simulink model "Two_Attitude_Estimation_ekf"  (R2021a)
settings: Solver=FixedStepAuto  StartTime=0.0  StopTime=200  FixedStep=Ts  RelTol=1e-5
values from neighbouring files (symbols this model uses):
  accel_filter_coef = [    0.0264    0.1405    0.3331    0.3331    0.1405    0.0264]    [quad_params_ekf.m]
  g = ref_acc(3)    [ekf_measurement_jacobian.m]    (also in quad_params_ekf.m = 9.81)
  gyro_filter_den = [ 1.0000    2.2287    2.5245    1.5773    0.5410    0.0796]    [quad_params_ekf.m]
  gyro_filter_num = [ 0.2821    1.2725    2.4208    2.4208    1.2725    0.2821]    [quad_params_ekf.m]
  I = [     0.005831943165131                   0                   0 ... (first row only)    [quad_params_ekf.m]
  Kd_rates = [0.05,0.05,0.1]'    [quad_params_ekf.m]
  Kd_vel = [0.8,0.8,0.3]'    [quad_params_ekf.m]
  Ki_vel = [0.1,0.1,0.1]'    [quad_params_ekf.m]
  km = 1.2e-7    (= 1.2e-07)    [quad_params_ekf.m]
  Kp_att = [6,6,6]'    [quad_params_ekf.m]
  Kp_pos = [7,7,3]'    [quad_params_ekf.m]
  Kp_rates = [10,10,10]'    [quad_params_ekf.m]
  Kp_vel = [3,3,5]'    [quad_params_ekf.m]
  kt = 0.9e-5    (= 9e-06)    [quad_params_ekf.m]
  L = 0.2    [quad_params_ekf.m]
  m = 0.9272    [quad_params_ekf.m]
  P_init = 0.01*eye(7)    [quad_params_ekf.m]
  Q = diag([0.015,0.0150,0.0150,0.0150,0.001,0.001,0.001])    [quad_params_ekf.m]
  q_init = [1;0;0;0]    [quad_params_ekf.m]
  R = diag([0.35,0.35,0.35,0.05,0.05,0.05])    [quad_params_ekf.m]
  rate_p_max = 3.5    [quad_params_ekf.m]
  thrust_max = thrust_max_per_motor*4    (= 32)    [quad_params_ekf.m]
  thrust_max_per_motor = 8    [quad_params_ekf.m]
  tilt_max = pi/6    (= 0.523598775598)    [quad_params_ekf.m]
  TQ_max_per_motor = km*(w_max.^2)    [quad_params_ekf.m]
  Ts = 0.001    [ekf_process_jacobian.m]    (also in ekf_process_model.m; quad_params_ekf.m)
  Ts_IMU = 0.001    [quad_params_ekf.m]
  Vb_init = [0;0;0]    [quad_params_ekf.m]
  vel_xy_max = 15    [quad_params_ekf.m]
  vel_z_max = 10    [quad_params_ekf.m]
  wb_init = [0;0;0]    [quad_params_ekf.m]
  x_0 = [1 0 0 0 0 0 0]'    [quad_params_ekf.m]
  Xe_init = [0;0;0]    [quad_params_ekf.m]
undefined symbols (not defined in the file or in its folder): IMU, p, pm_0, sigbuilder_block, Vm_0, xme_0
libraries: aerolibutil x8, simulink_extras x8, sharedtransform x7, sharedutil x6, simulink x4, pid_lib x3, aerolibcommonsys x3, aerolibnavsys x2, dspstat3 x2, mspsensorlib x1, aerolibnav x1, dspmtrx3 x1
(part 4 of 4)

== system Two_Attitude_Estimation_ekf/Trajectory command/X ramp/ ramp on X ==
  Demux : Demux  Tag=STV Demux
      settings: DisplayOption=none
  FromWs : FromWorkspace  Tag=STV FromWs  VariableName=tuvar
      SigBuilderData=|
      | common.afterFinalStr = 'Extrapolate'
      | common.sampleTime = 0
      | dataSet(1).timeRange = [0 200]
      | dataSet(1).name = 'small_steps'
      | dataSet(2).timeRange = [0 200]
      | dataSet(2).name = 'zStairs_xyConstVEL'
      | dataSet(3).timeRange = [0 500]
      | dataSet(3).name = 'sineWaves'
      | dataSet(4).timeRange = [0 200]
      | dataSet(4).name = 'ZERO'
      | dataSet(5).timeRange = [0 5]
      | dataSet(5).name = 'SEARCH_P1'
      | sbobj.Name = 'Signal Builder'
      | sbobj.Groups(1).Name = 'small_steps'
      | sbobj.Groups(1).Signals(1).Name = 'Z'
      | sbobj.Groups(1).Signals(1).XData = [0 10 10.000001 20 20.000001 30 30.000001 55 200]
      | sbobj.Groups(1).Signals(1).YData = [0 0 2 2 2 2 2 2 2]
      | sbobj.Groups(1).Signals(2).Name = 'Y'
      | sbobj.Groups(1).Signals(2).XData = [0 10 10.000001 20 20.000001 30 30.000001 55 200]
      | sbobj.Groups(1).Signals(2).YData = [0 0 0 0 3 3 3 3 3]
      | sbobj.Groups(1).Signals(3).Name = 'X'
      | sbobj.Groups(1).Signals(3).XData = [0 10 10.000001 20 20.000001 30 30.000001 55 200]
      | sbobj.Groups(1).Signals(3).YData = [0 0 0 0 0 0 1 1 1]
      | sbobj.Groups(1).Signals(4).Name = 'Yaw'
      | sbobj.Groups(1).Signals(4).XData = [0 200]
      | sbobj.Groups(1).Signals(4).YData = [0 0]
      | sbobj.Groups(1).TimeRange = [0 200]
      | sbobj.Groups(2).Name = 'zStairs_xyConstVEL'
      | sbobj.Groups(2).Signals(1).Name = 'Z'
      | sbobj.Groups(2).Signals(1).XData = [0 10 10.000001 20 20.000001 30 30.000001 40 40.000001 55 200]
      | sbobj.Groups(2).Signals(1).YData = [0 0 1 1 2 2 1 1 0 0 0]
      | sbobj.Groups(2).Signals(2).Name = 'Y'
      | sbobj.Groups(2).Signals(2).XData = [0 10 10.000001 20 20.000001 30 30.000001 40 40.000001 55 200]
      | sbobj.Groups(2).Signals(2).YData = [0 1 1.0000001 2 2.0000001 3 3.0000001 4 4.0000001 5.5 20]
      | sbobj.Groups(2).Signals(3).Name = 'X'
      | sbobj.Groups(2).Signals(3).XData = [0 10 10.000001 20 20.000001 30 30.000001 40 40.000001 55 200]
      | sbobj.Groups(2).Signals(3).YData = [0 0.5 0.50000005 1 1.00000005 1.5 1.50000005 2 2.00000005 2.75 10]
      | sbobj.Groups(2).Signals(4).Name = 'Yaw'
      | sbobj.Groups(2).Signals(4).XData = [0 200]
      | sbobj.Groups(2).Signals(4).YData = [0 0]
      | sbobj.Groups(2).TimeRange = [0 200]
      | sbobj.Groups(3).Name = 'sineWaves'
      | sbobj.Groups(3).Signals(1).Name = 'Z'
      | sbobj.Groups(3).Signals(1).XData = [0 0.1 0.2 0.3 0.4 0.5 0.6 0.7 0.8 0.9 1 1.1 ... (5001 elements, 1x5001)]
      | sbobj.Groups(3).Signals(1).YData = [0 0.0314107325553 0.0627904665622 0.0941082340641 0.125333128258 0.156434333994 0.18738115819 0.218143060119 0.248689681547 0.278990876699 0.309016742004 0.338737645607 ... (5001 elements, 1x5001)]
      | sbobj.Groups(3).Signals(2).Name = 'Y'
      | sbobj.Groups(3).Signals(2).XData = [0 0.1 0.2 0.3 0.4 0.5 0.6 0.7 0.8 0.9 1 1.1 ... (5001 elements, 1x5001)]
      | sbobj.Groups(3).Signals(2).YData = [0 0.01 0.02 0.03 0.04 0.05 0.06 0.07 0.08 0.09 0.1 0.11 ... (5001 elements, 1x5001)]
      | sbobj.Groups(3).Signals(3).Name = 'X'
      | sbobj.Groups(3).Signals(3).XData = [0 0.1 0.2 0.3 0.4 0.5 0.6 0.7 0.8 0.9 1 1.1 ... (5001 elements, 1x5001)]
      | sbobj.Groups(3).Signals(3).YData = [0 0.0157073040455 0.0314107325553 0.04710641095 0.0627904665622 0.0784590295926 0.0941082340641 0.109734218776 0.125333128258 0.140901113717 0.156434333994 0.171928956505 ... (5001 elements, 1x5001)]
      | sbobj.Groups(3).Signals(4).Name = 'Yaw'
      | sbobj.Groups(3).Signals(4).XData = [0 500]
      | sbobj.Groups(3).Signals(4).YData = [0 0]
      | sbobj.Groups(3).TimeRange = [0 500]
      | sbobj.Groups(4).Name = 'ZERO'
      | sbobj.Groups(4).Signals(1).Name = 'Z'
      | sbobj.Groups(4).Signals(1).XData = [0 200]
      | sbobj.Groups(4).Signals(1).YData = [0 0]
      | sbobj.Groups(4).Signals(2).Name = 'Y'
      | sbobj.Groups(4).Signals(2).XData = [0 200]
      | sbobj.Groups(4).Signals(2).YData = [0 0]
      | sbobj.Groups(4).Signals(3).Name = 'X'
      | sbobj.Groups(4).Signals(3).XData = [0 200]
      | sbobj.Groups(4).Signals(3).YData = [0 0]
      | sbobj.Groups(4).Signals(4).Name = 'Yaw'
      | sbobj.Groups(4).Signals(4).XData = [0 200]
      | sbobj.Groups(4).Signals(4).YData = [0 0]
      | sbobj.Groups(4).TimeRange = [0 200]
      | sbobj.Groups(5).Name = 'SEARCH_P1'
      | sbobj.Groups(5).Signals(1).Name = 'Z'
      | sbobj.Groups(5).Signals(1).XData = [0 5]
      | sbobj.Groups(5).Signals(1).YData = [0 0]
      | sbobj.Groups(5).Signals(2).Name = 'Y'
      | sbobj.Groups(5).Signals(2).XData = [0 5]
      | sbobj.Groups(5).Signals(2).YData = [0 0]
      | sbobj.Groups(5).Signals(3).Name = 'X'
      | sbobj.Groups(5).Signals(3).XData = [0 0.2 2 3 5]
      | sbobj.Groups(5).Signals(3).YData = [0 0 1 1 0]
      | sbobj.Groups(5).Signals(4).Name = 'Yaw'
      | sbobj.Groups(5).Signals(4).XData = [0 5]
      | sbobj.Groups(5).Signals(4).YData = [0 0]
      | sbobj.Groups(5).TimeRange = [0 5]
  Z : Outport  VectorParamsAs1DForOutWhenUnconnected=off
  Y : Outport  Tag=STV Outport  Port=2  VectorParamsAs1DForOutWhenUnconnected=off
  X : Outport  Tag=STV Outport  Port=3  VectorParamsAs1DForOutWhenUnconnected=off
  Yaw : Outport  Tag=STV Outport  Port=4
  wires:
  Demux/4 -> Yaw/1
  Demux/3 -> X/1
  Demux/2 -> Y/1
  FromWs/1 -> Demux/1
  Demux/1 -> Z/1

== system Two_Attitude_Estimation_ekf/Trajectory command/X square/sine wave on X ==
  Demux : Demux  Tag=STV Demux
      settings: DisplayOption=none
  FromWs : FromWorkspace  Tag=STV FromWs  VariableName=tuvar
      SigBuilderData=|
      | common.afterFinalStr = 'Extrapolate'
      | common.sampleTime = 0
      | dataSet(1).timeRange = [0 200]
      | dataSet(1).name = 'small_steps'
      | dataSet(2).timeRange = [0 200]
      | dataSet(2).name = 'zStairs_xyConstVEL'
      | dataSet(3).timeRange = [0 500]
      | dataSet(3).name = 'sineWaves'
      | dataSet(4).timeRange = [0 200]
      | dataSet(4).name = 'ZERO'
      | dataSet(5).timeRange = [0 20]
      | dataSet(5).name = 'SEARCH_P1'
      | sbobj.Name = 'Signal Builder'
      | sbobj.Groups(1).Name = 'small_steps'
      | sbobj.Groups(1).Signals(1).Name = 'Z'
      | sbobj.Groups(1).Signals(1).XData = [0 10 10.000001 20 20.000001 30 30.000001 55 200]
      | sbobj.Groups(1).Signals(1).YData = [0 0 2 2 2 2 2 2 2]
      | sbobj.Groups(1).Signals(2).Name = 'Y'
      | sbobj.Groups(1).Signals(2).XData = [0 10 10.000001 20 20.000001 30 30.000001 55 200]
      | sbobj.Groups(1).Signals(2).YData = [0 0 0 0 3 3 3 3 3]
      | sbobj.Groups(1).Signals(3).Name = 'X'
      | sbobj.Groups(1).Signals(3).XData = [0 10 10.000001 20 20.000001 30 30.000001 55 200]
      | sbobj.Groups(1).Signals(3).YData = [0 0 0 0 0 0 1 1 1]
      | sbobj.Groups(1).Signals(4).Name = 'Yaw'
      | sbobj.Groups(1).Signals(4).XData = [0 200]
      | sbobj.Groups(1).Signals(4).YData = [0 0]
      | sbobj.Groups(1).TimeRange = [0 200]
      | sbobj.Groups(2).Name = 'zStairs_xyConstVEL'
      | sbobj.Groups(2).Signals(1).Name = 'Z'
      | sbobj.Groups(2).Signals(1).XData = [0 10 10.000001 20 20.000001 30 30.000001 40 40.000001 55 200]
      | sbobj.Groups(2).Signals(1).YData = [0 0 1 1 2 2 1 1 0 0 0]
      | sbobj.Groups(2).Signals(2).Name = 'Y'
      | sbobj.Groups(2).Signals(2).XData = [0 10 10.000001 20 20.000001 30 30.000001 40 40.000001 55 200]
      | sbobj.Groups(2).Signals(2).YData = [0 1 1.0000001 2 2.0000001 3 3.0000001 4 4.0000001 5.5 20]
      | sbobj.Groups(2).Signals(3).Name = 'X'
      | sbobj.Groups(2).Signals(3).XData = [0 10 10.000001 20 20.000001 30 30.000001 40 40.000001 55 200]
      | sbobj.Groups(2).Signals(3).YData = [0 0.5 0.50000005 1 1.00000005 1.5 1.50000005 2 2.00000005 2.75 10]
      | sbobj.Groups(2).Signals(4).Name = 'Yaw'
      | sbobj.Groups(2).Signals(4).XData = [0 200]
      | sbobj.Groups(2).Signals(4).YData = [0 0]
      | sbobj.Groups(2).TimeRange = [0 200]
      | sbobj.Groups(3).Name = 'sineWaves'
      | sbobj.Groups(3).Signals(1).Name = 'Z'
      | sbobj.Groups(3).Signals(1).XData = [0 0.1 0.2 0.3 0.4 0.5 0.6 0.7 0.8 0.9 1 1.1 ... (5001 elements, 1x5001)]
      | sbobj.Groups(3).Signals(1).YData = [0 0.0314107325553 0.0627904665622 0.0941082340641 0.125333128258 0.156434333994 0.18738115819 0.218143060119 0.248689681547 0.278990876699 0.309016742004 0.338737645607 ... (5001 elements, 1x5001)]
      | sbobj.Groups(3).Signals(2).Name = 'Y'
      | sbobj.Groups(3).Signals(2).XData = [0 0.1 0.2 0.3 0.4 0.5 0.6 0.7 0.8 0.9 1 1.1 ... (5001 elements, 1x5001)]
      | sbobj.Groups(3).Signals(2).YData = [0 0.01 0.02 0.03 0.04 0.05 0.06 0.07 0.08 0.09 0.1 0.11 ... (5001 elements, 1x5001)]
      | sbobj.Groups(3).Signals(3).Name = 'X'
      | sbobj.Groups(3).Signals(3).XData = [0 0.1 0.2 0.3 0.4 0.5 0.6 0.7 0.8 0.9 1 1.1 ... (5001 elements, 1x5001)]
      | sbobj.Groups(3).Signals(3).YData = [0 0.0157073040455 0.0314107325553 0.04710641095 0.0627904665622 0.0784590295926 0.0941082340641 0.109734218776 0.125333128258 0.140901113717 0.156434333994 0.171928956505 ... (5001 elements, 1x5001)]
      | sbobj.Groups(3).Signals(4).Name = 'Yaw'
      | sbobj.Groups(3).Signals(4).XData = [0 500]
      | sbobj.Groups(3).Signals(4).YData = [0 0]
      | sbobj.Groups(3).TimeRange = [0 500]
      | sbobj.Groups(4).Name = 'ZERO'
      | sbobj.Groups(4).Signals(1).Name = 'Z'
      | sbobj.Groups(4).Signals(1).XData = [0 200]
      | sbobj.Groups(4).Signals(1).YData = [0 0]
      | sbobj.Groups(4).Signals(2).Name = 'Y'
      | sbobj.Groups(4).Signals(2).XData = [0 200]
      | sbobj.Groups(4).Signals(2).YData = [0 0]
      | sbobj.Groups(4).Signals(3).Name = 'X'
      | sbobj.Groups(4).Signals(3).XData = [0 200]
      | sbobj.Groups(4).Signals(3).YData = [0 0]
      | sbobj.Groups(4).Signals(4).Name = 'Yaw'
      | sbobj.Groups(4).Signals(4).XData = [0 200]
      | sbobj.Groups(4).Signals(4).YData = [0 0]
      | sbobj.Groups(4).TimeRange = [0 200]
      | sbobj.Groups(5).Name = 'SEARCH_P1'
      | sbobj.Groups(5).Signals(1).Name = 'Z'
      | sbobj.Groups(5).Signals(1).XData = [0 9.9 20]
      | sbobj.Groups(5).Signals(1).YData = [0 0 0]
      | sbobj.Groups(5).Signals(2).Name = 'Y'
      | sbobj.Groups(5).Signals(2).XData = [0 20]
      | sbobj.Groups(5).Signals(2).YData = [0 0]
      | sbobj.Groups(5).Signals(3).Name = 'X'
      | sbobj.Groups(5).Signals(3).XData = [0 5 5 10 10 15 15 20]
      | sbobj.Groups(5).Signals(3).YData = [0.2 0.2 -0.2 -0.2 0.2 0.2 -0.2 -0.2]
      | sbobj.Groups(5).Signals(4).Name = 'Yaw'
      | sbobj.Groups(5).Signals(4).XData = [0 20]
      | sbobj.Groups(5).Signals(4).YData = [0 0]
      | sbobj.Groups(5).TimeRange = [0 20]
  Z : Outport  VectorParamsAs1DForOutWhenUnconnected=off
  Y : Outport  Tag=STV Outport  Port=2  VectorParamsAs1DForOutWhenUnconnected=off
  X : Outport  Tag=STV Outport  Port=3  VectorParamsAs1DForOutWhenUnconnected=off
  Yaw : Outport  Tag=STV Outport  Port=4
  wires:
  Demux/4 -> Yaw/1
  Demux/3 -> X/1
  Demux/2 -> Y/1
  FromWs/1 -> Demux/1
  Demux/1 -> Z/1

== system Two_Attitude_Estimation_ekf/Trajectory command/Y Sine/sine wave on Y ==
  Demux : Demux  Tag=STV Demux
      settings: DisplayOption=none
  FromWs : FromWorkspace  Tag=STV FromWs  VariableName=tuvar
      SigBuilderData=|
      | common.afterFinalStr = 'Extrapolate'
      | common.sampleTime = 0
      | dataSet(1).timeRange = [0 200]
      | dataSet(1).name = 'small_steps'
      | dataSet(2).timeRange = [0 200]
      | dataSet(2).name = 'zStairs_xyConstVEL'
      | dataSet(3).timeRange = [0 500]
      | dataSet(3).name = 'sineWaves'
      | dataSet(4).timeRange = [0 200]
      | dataSet(4).name = 'ZERO'
      | dataSet(5).timeRange = [0 200]
      | dataSet(5).name = 'SEARCH_P1'
      | sbobj.Name = 'Signal Builder'
      | sbobj.Groups(1).Name = 'small_steps'
      | sbobj.Groups(1).Signals(1).Name = 'Z'
      | sbobj.Groups(1).Signals(1).XData = [0 10 10.000001 20 20.000001 30 30.000001 55 200]
      | sbobj.Groups(1).Signals(1).YData = [0 0 2 2 2 2 2 2 2]
      | sbobj.Groups(1).Signals(2).Name = 'Y'
      | sbobj.Groups(1).Signals(2).XData = [0 10 10.000001 20 20.000001 30 30.000001 55 200]
      | sbobj.Groups(1).Signals(2).YData = [0 0 0 0 3 3 3 3 3]
      | sbobj.Groups(1).Signals(3).Name = 'X'
      | sbobj.Groups(1).Signals(3).XData = [0 10 10.000001 20 20.000001 30 30.000001 55 200]
      | sbobj.Groups(1).Signals(3).YData = [0 0 0 0 0 0 1 1 1]
      | sbobj.Groups(1).Signals(4).Name = 'Yaw'
      | sbobj.Groups(1).Signals(4).XData = [0 200]
      | sbobj.Groups(1).Signals(4).YData = [0 0]
      | sbobj.Groups(1).TimeRange = [0 200]
      | sbobj.Groups(2).Name = 'zStairs_xyConstVEL'
      | sbobj.Groups(2).Signals(1).Name = 'Z'
      | sbobj.Groups(2).Signals(1).XData = [0 10 10.000001 20 20.000001 30 30.000001 40 40.000001 55 200]
      | sbobj.Groups(2).Signals(1).YData = [0 0 1 1 2 2 1 1 0 0 0]
      | sbobj.Groups(2).Signals(2).Name = 'Y'
      | sbobj.Groups(2).Signals(2).XData = [0 10 10.000001 20 20.000001 30 30.000001 40 40.000001 55 200]
      | sbobj.Groups(2).Signals(2).YData = [0 1 1.0000001 2 2.0000001 3 3.0000001 4 4.0000001 5.5 20]
      | sbobj.Groups(2).Signals(3).Name = 'X'
      | sbobj.Groups(2).Signals(3).XData = [0 10 10.000001 20 20.000001 30 30.000001 40 40.000001 55 200]
      | sbobj.Groups(2).Signals(3).YData = [0 0.5 0.50000005 1 1.00000005 1.5 1.50000005 2 2.00000005 2.75 10]
      | sbobj.Groups(2).Signals(4).Name = 'Yaw'
      | sbobj.Groups(2).Signals(4).XData = [0 200]
      | sbobj.Groups(2).Signals(4).YData = [0 0]
      | sbobj.Groups(2).TimeRange = [0 200]
      | sbobj.Groups(3).Name = 'sineWaves'
      | sbobj.Groups(3).Signals(1).Name = 'Z'
      | sbobj.Groups(3).Signals(1).XData = [0 0.1 0.2 0.3 0.4 0.5 0.6 0.7 0.8 0.9 1 1.1 ... (5001 elements, 1x5001)]
      | sbobj.Groups(3).Signals(1).YData = [0 0.0314107325553 0.0627904665622 0.0941082340641 0.125333128258 0.156434333994 0.18738115819 0.218143060119 0.248689681547 0.278990876699 0.309016742004 0.338737645607 ... (5001 elements, 1x5001)]
      | sbobj.Groups(3).Signals(2).Name = 'Y'
      | sbobj.Groups(3).Signals(2).XData = [0 0.1 0.2 0.3 0.4 0.5 0.6 0.7 0.8 0.9 1 1.1 ... (5001 elements, 1x5001)]
      | sbobj.Groups(3).Signals(2).YData = [0 0.01 0.02 0.03 0.04 0.05 0.06 0.07 0.08 0.09 0.1 0.11 ... (5001 elements, 1x5001)]
      | sbobj.Groups(3).Signals(3).Name = 'X'
      | sbobj.Groups(3).Signals(3).XData = [0 0.1 0.2 0.3 0.4 0.5 0.6 0.7 0.8 0.9 1 1.1 ... (5001 elements, 1x5001)]
      | sbobj.Groups(3).Signals(3).YData = [0 0.0157073040455 0.0314107325553 0.04710641095 0.0627904665622 0.0784590295926 0.0941082340641 0.109734218776 0.125333128258 0.140901113717 0.156434333994 0.171928956505 ... (5001 elements, 1x5001)]
      | sbobj.Groups(3).Signals(4).Name = 'Yaw'
      | sbobj.Groups(3).Signals(4).XData = [0 500]
      | sbobj.Groups(3).Signals(4).YData = [0 0]
      | sbobj.Groups(3).TimeRange = [0 500]
      | sbobj.Groups(4).Name = 'ZERO'
      | sbobj.Groups(4).Signals(1).Name = 'Z'
      | sbobj.Groups(4).Signals(1).XData = [0 200]
      | sbobj.Groups(4).Signals(1).YData = [0 0]
      | sbobj.Groups(4).Signals(2).Name = 'Y'
      | sbobj.Groups(4).Signals(2).XData = [0 200]
      | sbobj.Groups(4).Signals(2).YData = [0 0]
      | sbobj.Groups(4).Signals(3).Name = 'X'
      | sbobj.Groups(4).Signals(3).XData = [0 200]
      | sbobj.Groups(4).Signals(3).YData = [0 0]
      | sbobj.Groups(4).Signals(4).Name = 'Yaw'
      | sbobj.Groups(4).Signals(4).XData = [0 200]
      | sbobj.Groups(4).Signals(4).YData = [0 0]
      | sbobj.Groups(4).TimeRange = [0 200]
      | sbobj.Groups(5).Name = 'SEARCH_P1'
      | sbobj.Groups(5).Signals(1).Name = 'Z'
      | sbobj.Groups(5).Signals(1).XData = [0 9.9 200]
      | sbobj.Groups(5).Signals(1).YData = [0 0 0]
      | sbobj.Groups(5).Signals(2).Name = 'Y'
      | sbobj.Groups(5).Signals(2).XData = [0 0.689655172414 1.37931034483 2.06896551724 2.75862068966 3.44827586207 4.13793103448 4.8275862069 5.51724137931 6.20689655172 6.89655172414 7.58620689655 ... (291 elements, 1x291)]
      | sbobj.Groups(5).Signals(2).YData = [0 0.214970440211 0.41988910156 0.605174215194 0.762162055128 0.883512044446 0.963549992519 0.998533413851 0.986826522542 0.928976719817 0.827688998157 0.687699458853 ... (291 elements, 1x291)]
      | sbobj.Groups(5).Signals(3).Name = 'X'
      | sbobj.Groups(5).Signals(3).XData = [0 9.9 200]
      | sbobj.Groups(5).Signals(3).YData = [0 0 0]
      | sbobj.Groups(5).Signals(4).Name = 'Yaw'
      | sbobj.Groups(5).Signals(4).XData = [0 200]
      | sbobj.Groups(5).Signals(4).YData = [0 0]
      | sbobj.Groups(5).TimeRange = [0 200]
  Z : Outport  VectorParamsAs1DForOutWhenUnconnected=off
  Y : Outport  Tag=STV Outport  Port=2  VectorParamsAs1DForOutWhenUnconnected=off
  X : Outport  Tag=STV Outport  Port=3  VectorParamsAs1DForOutWhenUnconnected=off
  Yaw : Outport  Tag=STV Outport  Port=4
  wires:
  Demux/4 -> Yaw/1
  Demux/3 -> X/1
  Demux/2 -> Y/1
  FromWs/1 -> Demux/1
  Demux/1 -> Z/1

== system Two_Attitude_Estimation_ekf/Trajectory command/Y ramp/square on Y ==
  Demux : Demux  Tag=STV Demux
      settings: DisplayOption=none
  FromWs : FromWorkspace  Tag=STV FromWs  VariableName=tuvar
      SigBuilderData=|
      | common.afterFinalStr = 'Extrapolate'
      | common.sampleTime = 0
      | dataSet(1).timeRange = [0 200]
      | dataSet(1).name = 'small_steps'
      | dataSet(2).timeRange = [0 200]
      | dataSet(2).name = 'zStairs_xyConstVEL'
      | dataSet(3).timeRange = [0 500]
      | dataSet(3).name = 'sineWaves'
      | dataSet(4).timeRange = [0 200]
      | dataSet(4).name = 'ZERO'
      | dataSet(5).timeRange = [0 20]
      | dataSet(5).name = 'SEARCH_P1'
      | sbobj.Name = 'Signal Builder'
      | sbobj.Groups(1).Name = 'small_steps'
      | sbobj.Groups(1).Signals(1).Name = 'Z'
      | sbobj.Groups(1).Signals(1).XData = [0 10 10.000001 20 20.000001 30 30.000001 55 200]
      | sbobj.Groups(1).Signals(1).YData = [0 0 2 2 2 2 2 2 2]
      | sbobj.Groups(1).Signals(2).Name = 'Y'
      | sbobj.Groups(1).Signals(2).XData = [0 10 10.000001 20 20.000001 30 30.000001 55 200]
      | sbobj.Groups(1).Signals(2).YData = [0 0 0 0 3 3 3 3 3]
      | sbobj.Groups(1).Signals(3).Name = 'X'
      | sbobj.Groups(1).Signals(3).XData = [0 10 10.000001 20 20.000001 30 30.000001 55 200]
      | sbobj.Groups(1).Signals(3).YData = [0 0 0 0 0 0 1 1 1]
      | sbobj.Groups(1).Signals(4).Name = 'Yaw'
      | sbobj.Groups(1).Signals(4).XData = [0 200]
      | sbobj.Groups(1).Signals(4).YData = [0 0]
      | sbobj.Groups(1).TimeRange = [0 200]
      | sbobj.Groups(2).Name = 'zStairs_xyConstVEL'
      | sbobj.Groups(2).Signals(1).Name = 'Z'
      | sbobj.Groups(2).Signals(1).XData = [0 10 10.000001 20 20.000001 30 30.000001 40 40.000001 55 200]
      | sbobj.Groups(2).Signals(1).YData = [0 0 1 1 2 2 1 1 0 0 0]
      | sbobj.Groups(2).Signals(2).Name = 'Y'
      | sbobj.Groups(2).Signals(2).XData = [0 10 10.000001 20 20.000001 30 30.000001 40 40.000001 55 200]
      | sbobj.Groups(2).Signals(2).YData = [0 1 1.0000001 2 2.0000001 3 3.0000001 4 4.0000001 5.5 20]
      | sbobj.Groups(2).Signals(3).Name = 'X'
      | sbobj.Groups(2).Signals(3).XData = [0 10 10.000001 20 20.000001 30 30.000001 40 40.000001 55 200]
      | sbobj.Groups(2).Signals(3).YData = [0 0.5 0.50000005 1 1.00000005 1.5 1.50000005 2 2.00000005 2.75 10]
      | sbobj.Groups(2).Signals(4).Name = 'Yaw'
      | sbobj.Groups(2).Signals(4).XData = [0 200]
      | sbobj.Groups(2).Signals(4).YData = [0 0]
      | sbobj.Groups(2).TimeRange = [0 200]
      | sbobj.Groups(3).Name = 'sineWaves'
      | sbobj.Groups(3).Signals(1).Name = 'Z'
      | sbobj.Groups(3).Signals(1).XData = [0 0.1 0.2 0.3 0.4 0.5 0.6 0.7 0.8 0.9 1 1.1 ... (5001 elements, 1x5001)]
      | sbobj.Groups(3).Signals(1).YData = [0 0.0314107325553 0.0627904665622 0.0941082340641 0.125333128258 0.156434333994 0.18738115819 0.218143060119 0.248689681547 0.278990876699 0.309016742004 0.338737645607 ... (5001 elements, 1x5001)]
      | sbobj.Groups(3).Signals(2).Name = 'Y'
      | sbobj.Groups(3).Signals(2).XData = [0 0.1 0.2 0.3 0.4 0.5 0.6 0.7 0.8 0.9 1 1.1 ... (5001 elements, 1x5001)]
      | sbobj.Groups(3).Signals(2).YData = [0 0.01 0.02 0.03 0.04 0.05 0.06 0.07 0.08 0.09 0.1 0.11 ... (5001 elements, 1x5001)]
      | sbobj.Groups(3).Signals(3).Name = 'X'
      | sbobj.Groups(3).Signals(3).XData = [0 0.1 0.2 0.3 0.4 0.5 0.6 0.7 0.8 0.9 1 1.1 ... (5001 elements, 1x5001)]
      | sbobj.Groups(3).Signals(3).YData = [0 0.0157073040455 0.0314107325553 0.04710641095 0.0627904665622 0.0784590295926 0.0941082340641 0.109734218776 0.125333128258 0.140901113717 0.156434333994 0.171928956505 ... (5001 elements, 1x5001)]
      | sbobj.Groups(3).Signals(4).Name = 'Yaw'
      | sbobj.Groups(3).Signals(4).XData = [0 500]
      | sbobj.Groups(3).Signals(4).YData = [0 0]
      | sbobj.Groups(3).TimeRange = [0 500]
      | sbobj.Groups(4).Name = 'ZERO'
      | sbobj.Groups(4).Signals(1).Name = 'Z'
      | sbobj.Groups(4).Signals(1).XData = [0 200]
      | sbobj.Groups(4).Signals(1).YData = [0 0]
      | sbobj.Groups(4).Signals(2).Name = 'Y'
      | sbobj.Groups(4).Signals(2).XData = [0 200]
      | sbobj.Groups(4).Signals(2).YData = [0 0]
      | sbobj.Groups(4).Signals(3).Name = 'X'
      | sbobj.Groups(4).Signals(3).XData = [0 200]
      | sbobj.Groups(4).Signals(3).YData = [0 0]
      | sbobj.Groups(4).Signals(4).Name = 'Yaw'
      | sbobj.Groups(4).Signals(4).XData = [0 200]
      | sbobj.Groups(4).Signals(4).YData = [0 0]
      | sbobj.Groups(4).TimeRange = [0 200]
      | sbobj.Groups(5).Name = 'SEARCH_P1'
      | sbobj.Groups(5).Signals(1).Name = 'Z'
      | sbobj.Groups(5).Signals(1).XData = [0 9.9 20]
      | sbobj.Groups(5).Signals(1).YData = [0 0 0]
      | sbobj.Groups(5).Signals(2).Name = 'Y'
      | sbobj.Groups(5).Signals(2).XData = [0 5 7 10 12 15 17 20]
      | sbobj.Groups(5).Signals(2).YData = [0.2 0.2 -0.2 -0.2 0.2 0.2 -0.2 -0.2]
      | sbobj.Groups(5).Signals(3).Name = 'X'
      | sbobj.Groups(5).Signals(3).XData = [0 9.9 20]
      | sbobj.Groups(5).Signals(3).YData = [0 0 0]
      | sbobj.Groups(5).Signals(4).Name = 'Yaw'
      | sbobj.Groups(5).Signals(4).XData = [0 20]
      | sbobj.Groups(5).Signals(4).YData = [0 0]
      | sbobj.Groups(5).TimeRange = [0 20]
  Z : Outport  VectorParamsAs1DForOutWhenUnconnected=off
  Y : Outport  Tag=STV Outport  Port=2  VectorParamsAs1DForOutWhenUnconnected=off
  X : Outport  Tag=STV Outport  Port=3  VectorParamsAs1DForOutWhenUnconnected=off
  Yaw : Outport  Tag=STV Outport  Port=4
  wires:
  Demux/4 -> Yaw/1
  Demux/3 -> X/1
  Demux/2 -> Y/1
  FromWs/1 -> Demux/1
  Demux/1 -> Z/1

== system Two_Attitude_Estimation_ekf/Trajectory command/Yaw Sine/yaw ==
  Demux : Demux  Tag=STV Demux
      settings: DisplayOption=none
  FromWs : FromWorkspace  Tag=STV FromWs  VariableName=tuvar
      SigBuilderData=|
      | common.afterFinalStr = 'Extrapolate'
      | common.sampleTime = 0
      | dataSet(1).timeRange = [0 200]
      | dataSet(1).name = 'small_steps'
      | dataSet(2).timeRange = [0 200]
      | dataSet(2).name = 'zStairs_xyConstVEL'
      | dataSet(3).timeRange = [0 500]
      | dataSet(3).name = 'sineWaves'
      | dataSet(4).timeRange = [0 200]
      | dataSet(4).name = 'ZERO'
      | dataSet(5).timeRange = [0 200]
      | dataSet(5).name = 'SEARCH_P1'
      | sbobj.Name = 'Signal Builder'
      | sbobj.Groups(1).Name = 'small_steps'
      | sbobj.Groups(1).Signals(1).Name = 'Z'
      | sbobj.Groups(1).Signals(1).XData = [0 10 10.000001 20 20.000001 30 30.000001 55 200]
      | sbobj.Groups(1).Signals(1).YData = [0 0 2 2 2 2 2 2 2]
      | sbobj.Groups(1).Signals(2).Name = 'Y'
      | sbobj.Groups(1).Signals(2).XData = [0 10 10.000001 20 20.000001 30 30.000001 55 200]
      | sbobj.Groups(1).Signals(2).YData = [0 0 0 0 3 3 3 3 3]
      | sbobj.Groups(1).Signals(3).Name = 'X'
      | sbobj.Groups(1).Signals(3).XData = [0 10 10.000001 20 20.000001 30 30.000001 55 200]
      | sbobj.Groups(1).Signals(3).YData = [0 0 0 0 0 0 1 1 1]
      | sbobj.Groups(1).Signals(4).Name = 'Yaw'
      | sbobj.Groups(1).Signals(4).XData = [0 200]
      | sbobj.Groups(1).Signals(4).YData = [0 0]
      | sbobj.Groups(1).TimeRange = [0 200]
      | sbobj.Groups(2).Name = 'zStairs_xyConstVEL'
      | sbobj.Groups(2).Signals(1).Name = 'Z'
      | sbobj.Groups(2).Signals(1).XData = [0 10 10.000001 20 20.000001 30 30.000001 40 40.000001 55 200]
      | sbobj.Groups(2).Signals(1).YData = [0 0 1 1 2 2 1 1 0 0 0]
      | sbobj.Groups(2).Signals(2).Name = 'Y'
      | sbobj.Groups(2).Signals(2).XData = [0 10 10.000001 20 20.000001 30 30.000001 40 40.000001 55 200]
      | sbobj.Groups(2).Signals(2).YData = [0 1 1.0000001 2 2.0000001 3 3.0000001 4 4.0000001 5.5 20]
      | sbobj.Groups(2).Signals(3).Name = 'X'
      | sbobj.Groups(2).Signals(3).XData = [0 10 10.000001 20 20.000001 30 30.000001 40 40.000001 55 200]
      | sbobj.Groups(2).Signals(3).YData = [0 0.5 0.50000005 1 1.00000005 1.5 1.50000005 2 2.00000005 2.75 10]
      | sbobj.Groups(2).Signals(4).Name = 'Yaw'
      | sbobj.Groups(2).Signals(4).XData = [0 200]
      | sbobj.Groups(2).Signals(4).YData = [0 0]
      | sbobj.Groups(2).TimeRange = [0 200]
      | sbobj.Groups(3).Name = 'sineWaves'
      | sbobj.Groups(3).Signals(1).Name = 'Z'
      | sbobj.Groups(3).Signals(1).XData = [0 0.1 0.2 0.3 0.4 0.5 0.6 0.7 0.8 0.9 1 1.1 ... (5001 elements, 1x5001)]
      | sbobj.Groups(3).Signals(1).YData = [0 0.0314107325553 0.0627904665622 0.0941082340641 0.125333128258 0.156434333994 0.18738115819 0.218143060119 0.248689681547 0.278990876699 0.309016742004 0.338737645607 ... (5001 elements, 1x5001)]
      | sbobj.Groups(3).Signals(2).Name = 'Y'
      | sbobj.Groups(3).Signals(2).XData = [0 0.1 0.2 0.3 0.4 0.5 0.6 0.7 0.8 0.9 1 1.1 ... (5001 elements, 1x5001)]
      | sbobj.Groups(3).Signals(2).YData = [0 0.01 0.02 0.03 0.04 0.05 0.06 0.07 0.08 0.09 0.1 0.11 ... (5001 elements, 1x5001)]
      | sbobj.Groups(3).Signals(3).Name = 'X'
      | sbobj.Groups(3).Signals(3).XData = [0 0.1 0.2 0.3 0.4 0.5 0.6 0.7 0.8 0.9 1 1.1 ... (5001 elements, 1x5001)]
      | sbobj.Groups(3).Signals(3).YData = [0 0.0157073040455 0.0314107325553 0.04710641095 0.0627904665622 0.0784590295926 0.0941082340641 0.109734218776 0.125333128258 0.140901113717 0.156434333994 0.171928956505 ... (5001 elements, 1x5001)]
      | sbobj.Groups(3).Signals(4).Name = 'Yaw'
      | sbobj.Groups(3).Signals(4).XData = [0 500]
      | sbobj.Groups(3).Signals(4).YData = [0 0]
      | sbobj.Groups(3).TimeRange = [0 500]
      | sbobj.Groups(4).Name = 'ZERO'
      | sbobj.Groups(4).Signals(1).Name = 'Z'
      | sbobj.Groups(4).Signals(1).XData = [0 200]
      | sbobj.Groups(4).Signals(1).YData = [0 0]
      | sbobj.Groups(4).Signals(2).Name = 'Y'
      | sbobj.Groups(4).Signals(2).XData = [0 200]
      | sbobj.Groups(4).Signals(2).YData = [0 0]
      | sbobj.Groups(4).Signals(3).Name = 'X'
      | sbobj.Groups(4).Signals(3).XData = [0 200]
      | sbobj.Groups(4).Signals(3).YData = [0 0]
      | sbobj.Groups(4).Signals(4).Name = 'Yaw'
      | sbobj.Groups(4).Signals(4).XData = [0 200]
      | sbobj.Groups(4).Signals(4).YData = [0 0]
      | sbobj.Groups(4).TimeRange = [0 200]
      | sbobj.Groups(5).Name = 'SEARCH_P1'
      | sbobj.Groups(5).Signals(1).Name = 'Z'
      | sbobj.Groups(5).Signals(1).XData = [0 9.9 200]
      | sbobj.Groups(5).Signals(1).YData = [0 0 0]
      | sbobj.Groups(5).Signals(2).Name = 'Y'
      | sbobj.Groups(5).Signals(2).XData = [0 200]
      | sbobj.Groups(5).Signals(2).YData = [0 0]
      | sbobj.Groups(5).Signals(3).Name = 'X'
      | sbobj.Groups(5).Signals(3).XData = [0 200]
      | sbobj.Groups(5).Signals(3).YData = [0 0]
      | sbobj.Groups(5).Signals(4).Name = 'Yaw'
      | sbobj.Groups(5).Signals(4).XData = [0 0.689655172414 1.37931034483 2.06896551724 2.75862068966 3.44827586207 4.13793103448 4.8275862069 5.51724137931 6.20689655172 6.89655172414 7.58620689655 ... (291 elements, 1x291)]
      | sbobj.Groups(5).Signals(4).YData = [0 0.644911320633 1.25966730468 1.81552264558 2.28648616538 2.65053613334 2.89064997756 2.99560024155 2.96047956762 2.78693015945 2.48306699447 2.06309837656 ... (291 elements, 1x291)]
      | sbobj.Groups(5).TimeRange = [0 200]
  Z : Outport  VectorParamsAs1DForOutWhenUnconnected=off
  Y : Outport  Tag=STV Outport  Port=2  VectorParamsAs1DForOutWhenUnconnected=off
  X : Outport  Tag=STV Outport  Port=3  VectorParamsAs1DForOutWhenUnconnected=off
  Yaw : Outport  Tag=STV Outport  Port=4
  wires:
  Demux/4 -> Yaw/1
  Demux/3 -> X/1
  Demux/2 -> Y/1
  FromWs/1 -> Demux/1
  Demux/1 -> Z/1

== system Two_Attitude_Estimation_ekf/Trajectory command/Yaw steps/yaw steps ==
  Demux : Demux  Tag=STV Demux
      settings: DisplayOption=none
  FromWs : FromWorkspace  Tag=STV FromWs  VariableName=tuvar
      SigBuilderData=|
      | common.afterFinalStr = 'Extrapolate'
      | common.sampleTime = 0
      | dataSet(1).timeRange = [0 200]
      | dataSet(1).name = 'small_steps'
      | dataSet(2).timeRange = [0 200]
      | dataSet(2).name = 'zStairs_xyConstVEL'
      | dataSet(3).timeRange = [0 500]
      | dataSet(3).name = 'sineWaves'
      | dataSet(4).timeRange = [0 200]
      | dataSet(4).name = 'ZERO'
      | dataSet(5).timeRange = [0 200]
      | dataSet(5).name = 'SEARCH_P1'
      | sbobj.Name = 'Signal Builder'
      | sbobj.Groups(1).Name = 'small_steps'
      | sbobj.Groups(1).Signals(1).Name = 'Z'
      | sbobj.Groups(1).Signals(1).XData = [0 10 10.000001 20 20.000001 30 30.000001 55 200]
      | sbobj.Groups(1).Signals(1).YData = [0 0 2 2 2 2 2 2 2]
      | sbobj.Groups(1).Signals(2).Name = 'Y'
      | sbobj.Groups(1).Signals(2).XData = [0 10 10.000001 20 20.000001 30 30.000001 55 200]
      | sbobj.Groups(1).Signals(2).YData = [0 0 0 0 3 3 3 3 3]
      | sbobj.Groups(1).Signals(3).Name = 'X'
      | sbobj.Groups(1).Signals(3).XData = [0 10 10.000001 20 20.000001 30 30.000001 55 200]
      | sbobj.Groups(1).Signals(3).YData = [0 0 0 0 0 0 1 1 1]
      | sbobj.Groups(1).Signals(4).Name = 'Yaw'
      | sbobj.Groups(1).Signals(4).XData = [0 200]
      | sbobj.Groups(1).Signals(4).YData = [0 0]
      | sbobj.Groups(1).TimeRange = [0 200]
      | sbobj.Groups(2).Name = 'zStairs_xyConstVEL'
      | sbobj.Groups(2).Signals(1).Name = 'Z'
      | sbobj.Groups(2).Signals(1).XData = [0 10 10.000001 20 20.000001 30 30.000001 40 40.000001 55 200]
      | sbobj.Groups(2).Signals(1).YData = [0 0 1 1 2 2 1 1 0 0 0]
      | sbobj.Groups(2).Signals(2).Name = 'Y'
      | sbobj.Groups(2).Signals(2).XData = [0 10 10.000001 20 20.000001 30 30.000001 40 40.000001 55 200]
      | sbobj.Groups(2).Signals(2).YData = [0 1 1.0000001 2 2.0000001 3 3.0000001 4 4.0000001 5.5 20]
      | sbobj.Groups(2).Signals(3).Name = 'X'
      | sbobj.Groups(2).Signals(3).XData = [0 10 10.000001 20 20.000001 30 30.000001 40 40.000001 55 200]
      | sbobj.Groups(2).Signals(3).YData = [0 0.5 0.50000005 1 1.00000005 1.5 1.50000005 2 2.00000005 2.75 10]
      | sbobj.Groups(2).Signals(4).Name = 'Yaw'
      | sbobj.Groups(2).Signals(4).XData = [0 200]
      | sbobj.Groups(2).Signals(4).YData = [0 0]
      | sbobj.Groups(2).TimeRange = [0 200]
      | sbobj.Groups(3).Name = 'sineWaves'
      | sbobj.Groups(3).Signals(1).Name = 'Z'
      | sbobj.Groups(3).Signals(1).XData = [0 0.1 0.2 0.3 0.4 0.5 0.6 0.7 0.8 0.9 1 1.1 ... (5001 elements, 1x5001)]
      | sbobj.Groups(3).Signals(1).YData = [0 0.0314107325553 0.0627904665622 0.0941082340641 0.125333128258 0.156434333994 0.18738115819 0.218143060119 0.248689681547 0.278990876699 0.309016742004 0.338737645607 ... (5001 elements, 1x5001)]
      | sbobj.Groups(3).Signals(2).Name = 'Y'
      | sbobj.Groups(3).Signals(2).XData = [0 0.1 0.2 0.3 0.4 0.5 0.6 0.7 0.8 0.9 1 1.1 ... (5001 elements, 1x5001)]
      | sbobj.Groups(3).Signals(2).YData = [0 0.01 0.02 0.03 0.04 0.05 0.06 0.07 0.08 0.09 0.1 0.11 ... (5001 elements, 1x5001)]
      | sbobj.Groups(3).Signals(3).Name = 'X'
      | sbobj.Groups(3).Signals(3).XData = [0 0.1 0.2 0.3 0.4 0.5 0.6 0.7 0.8 0.9 1 1.1 ... (5001 elements, 1x5001)]
      | sbobj.Groups(3).Signals(3).YData = [0 0.0157073040455 0.0314107325553 0.04710641095 0.0627904665622 0.0784590295926 0.0941082340641 0.109734218776 0.125333128258 0.140901113717 0.156434333994 0.171928956505 ... (5001 elements, 1x5001)]
      | sbobj.Groups(3).Signals(4).Name = 'Yaw'
      | sbobj.Groups(3).Signals(4).XData = [0 500]
      | sbobj.Groups(3).Signals(4).YData = [0 0]
      | sbobj.Groups(3).TimeRange = [0 500]
      | sbobj.Groups(4).Name = 'ZERO'
      | sbobj.Groups(4).Signals(1).Name = 'Z'
      | sbobj.Groups(4).Signals(1).XData = [0 200]
      | sbobj.Groups(4).Signals(1).YData = [0 0]
      | sbobj.Groups(4).Signals(2).Name = 'Y'
      | sbobj.Groups(4).Signals(2).XData = [0 200]
      | sbobj.Groups(4).Signals(2).YData = [0 0]
      | sbobj.Groups(4).Signals(3).Name = 'X'
      | sbobj.Groups(4).Signals(3).XData = [0 200]
      | sbobj.Groups(4).Signals(3).YData = [0 0]
      | sbobj.Groups(4).Signals(4).Name = 'Yaw'
      | sbobj.Groups(4).Signals(4).XData = [0 200]
      | sbobj.Groups(4).Signals(4).YData = [0 0]
      | sbobj.Groups(4).TimeRange = [0 200]
      | sbobj.Groups(5).Name = 'SEARCH_P1'
      | sbobj.Groups(5).Signals(1).Name = 'Z'
      | sbobj.Groups(5).Signals(1).XData = [0 9.9 200]
      | sbobj.Groups(5).Signals(1).YData = [0 0 0]
      | sbobj.Groups(5).Signals(2).Name = 'Y'
      | sbobj.Groups(5).Signals(2).XData = [0 200]
      | sbobj.Groups(5).Signals(2).YData = [0 0]
      | sbobj.Groups(5).Signals(3).Name = 'X'
      | sbobj.Groups(5).Signals(3).XData = [0 200]
      | sbobj.Groups(5).Signals(3).YData = [0 0]
      | sbobj.Groups(5).Signals(4).Name = 'Yaw'
      | sbobj.Groups(5).Signals(4).XData = [0 9.8 9.8 29.8 29.8 200]
      | sbobj.Groups(5).Signals(4).YData = [0 0 1.57 1.57 0.7854 0.7854]
      | sbobj.Groups(5).TimeRange = [0 200]
  Z : Outport  VectorParamsAs1DForOutWhenUnconnected=off
  Y : Outport  Tag=STV Outport  Port=2  VectorParamsAs1DForOutWhenUnconnected=off
  X : Outport  Tag=STV Outport  Port=3  VectorParamsAs1DForOutWhenUnconnected=off
  Yaw : Outport  Tag=STV Outport  Port=4
  wires:
  Demux/4 -> Yaw/1
  Demux/3 -> X/1
  Demux/2 -> Y/1
  FromWs/1 -> Demux/1
  Demux/1 -> Z/1

== system Two_Attitude_Estimation_ekf/Control allocation and motor control/Ideal Actuators with allocation/Control allocation/Subsystem ==
  w_per_sec : Inport
  Constant3 : Constant  Value=3.141592653589793
  Gain1 : Gain  Gain=2
  Product : Product  Inputs=*/
  RPS : Outport
  wires:
  Gain1/1 -> Product/2  "2PI"
  w_per_sec/1 -> Product/1
  Constant3/1 -> Gain1/1
  Product/1 -> RPS/1

== system Two_Attitude_Estimation_ekf/Control allocation and motor control/Ideal Actuators with allocation/Control allocation/W2_checker ==
  w2_CMD : Inport
  Assertion{,1..3} (4 alike) : Assertion
  Compare To Constant : simulink/Logic and Bit Operations/Compare To Constant  relop=>=  const=0  OutDataTypeStr=boolean
  Demux : Demux
  w2 : Outport  VectorParamsAs1DForOutWhenUnconnected=off
  wires:
  w2_CMD/1 -> w2/1, Compare To Constant/1
  Compare To Constant/1 -> Demux/1
  Demux/1 -> Assertion/1
  Demux/4 -> Assertion3/1
  Demux/3 -> Assertion2/1
  Demux/2 -> Assertion1/1

== system Two_Attitude_Estimation_ekf/Control allocation and motor control/Ideal Actuators with allocation/Perfect actuators/Motor Control ==
  w_CMD : Inport
  Demux : Demux
  Mux : Mux
  w CMD vs Actual : Scope  NumInputPorts=4
  w_MUX : Subsystem
  w : Outport  VectorParamsAs1DForOutWhenUnconnected=off
  wires:
  Demux/4 -> Mux/4
  Demux/3 -> Mux/3
  Demux/2 -> Mux/2
  Demux/1 -> Mux/1
  w_CMD/1 -> [W_CMD], Demux/1
  w_MUX/4(w4) -> w CMD vs Actual/4
  w_MUX/2(w2) -> w CMD vs Actual/2
  w_MUX/3(w3) -> w CMD vs Actual/3
  w_MUX/1(w1) -> w CMD vs Actual/1
  [W_CMD] -> w_MUX/1(W_CMD)
  Mux/1 -> w_MUX/2(W), w/1

== system Two_Attitude_Estimation_ekf/Quad with sensors/Integrate_quaternion/NORMLIZE_occasionally/Adjust_to_UNITY ==
  note: Every 10 seconds normalize
      | the quaternion to ensure it is a
      | UNIT quaternion
  qin : Inport
  Data Type Conversion : DataTypeConversion  OutDataTypeStr=double
  Detect Increase : simulink/Logic and Bit Operations/Detect Increase  vinit=0.0  OutDataTypeStr=boolean
  MATLAB Function : MATLAB Function  TreatAsAtomicUnit=on
  Pulse Generator : DiscretePulseGenerator  PulseType=Time based  Period=10  PulseWidth=50
  Scope : Scope
  q_unit : Outport
  wires:
  Pulse Generator/1 -> Detect Increase/1
  Detect Increase/1 -> Data Type Conversion/1
  MATLAB Function/1(q) -> q_unit/1
  Data Type Conversion/1 -> MATLAB Function/1(change_signal)
  qin/1 -> MATLAB Function/2(q_in)
  MATLAB Function/2(mag_of_q) -> Scope/1

== system Two_Attitude_Estimation_ekf/Quad_EOM/Integrate_quaternion/NORMLIZE_occasionally/Adjust_to_UNITY ==
  note: Every 10 seconds normalize
      | the quaternion to ensure it is a
      | UNIT quaternion
  qin : Inport
  Data Type Conversion : DataTypeConversion  OutDataTypeStr=double
  Detect Increase : simulink/Logic and Bit Operations/Detect Increase  vinit=0.0  OutDataTypeStr=boolean
  MATLAB Function : MATLAB Function  TreatAsAtomicUnit=on
  Pulse Generator : DiscretePulseGenerator  PulseType=Time based  Period=10  PulseWidth=50
  Scope : Scope
  q_unit : Outport
  wires:
  Pulse Generator/1 -> Detect Increase/1
  Detect Increase/1 -> Data Type Conversion/1
  MATLAB Function/1(q) -> q_unit/1
  Data Type Conversion/1 -> MATLAB Function/1(change_signal)
  qin/1 -> MATLAB Function/2(q_in)
  MATLAB Function/2(mag_of_q) -> Scope/1

== system Two_Attitude_Estimation_ekf/Sensors and preprocessing/IMU+altitude/Acc + Gyro/Acceleration Conversion ==
  acceleration : Inport  Unit=m/s^2
  Unit Conversion : UnitConversion
  inherit : Outport  VectorParamsAs1DForOutWhenUnconnected=off
  wires:
  Unit Conversion/1 -> inherit/1
  acceleration/1 -> Unit Conversion/1

== system Two_Attitude_Estimation_ekf/Sensors and preprocessing/IMU+altitude/Acc + Gyro/Three-axis Accelerometer ==
  Ab : Inport  Unit=m/s^2  PortDimensions=3
  p q r : Inport  Port=2  Unit=rad/s  PortDimensions=3
  pdot qdot rdot : Inport  Port=3  Unit=rad/s^2  PortDimensions=3
  CG : Inport  Port=4  Unit=m  PortDimensions=3
  g : Inport  Port=5  Unit=m/s^2  PortDimensions=3
  Disallow CGS : UnitConfiguration  UnitSystemsStr=English,SI,SI (extended)  AllowAllUnitSystems=off
  Dynamics : Subsystem
  Gain : Gain  Gain=[1 -1 1]  SaturateOnIntegerOverflow=on  OutDataTypeStr=Inherit: Same as input  ParamDataTypeStr=Inherit: Same as input
  Measurement bias : Constant  Value=a_bias
  Product : Product  Multiplication=Matrix(*)  SaturateOnIntegerOverflow=on  OutDataTypeStr=Inherit: Same as first input
  Random bias : aerolibcommonsys/Tunable White Noise  pwr=a_pow  Ts=a_Ts  seed=a_seeds
      settings: SourceProductBaseCode=AE
  Reshape1 : Reshape
  Saturation : Saturate  UpperLimit=a_sath  LowerLimit=a_satl
  Scale factors & Cross-coupling errors : Constant  Value=a_sf_cc
  Scope{,1..3} (4 alike) : Scope
  Sum : Sum  Inputs=+-++  SaturateOnIntegerOverflow=on
  Sum1 : Sum  Inputs=|++  SaturateOnIntegerOverflow=on
  Sum4 : Sum  Inputs=++|  SaturateOnIntegerOverflow=on
  Sum7 : Sum  Inputs=|+-  SaturateOnIntegerOverflow=on
  Zero-Order Hold{,1..4} (5 alike) : ZeroOrderHold  SampleTime=a_Ts
  w x (w x d) : Subsystem
  wdot x d : sharedutil/3x3 Cross Product  aMode=aMode
      settings: SourceProductBaseCode=AE,PW,DR,MT,UV,VE
  wl_ins : Constant  Value=acc
  Ameas : Outport  Unit=m/s^2  PortDimensions=3  VectorParamsAs1DForOutWhenUnconnected=off
  wires:
  Zero-Order Hold4/1 -> Sum7/1
  Zero-Order Hold3/1 -> wdot x d/1
  Zero-Order Hold/1 -> w x (w x d)/1("p q r ")
  Zero-Order Hold2/1 -> Scope1/1, Sum/2
  Zero-Order Hold1/1 -> Sum/1
  g/1 -> Zero-Order Hold2/1
  Gain/1 -> wdot x d/2, w x (w x d)/2(distance)
  wl_ins/1 -> Sum7/2
  Sum7/1 -> Gain/1
  Dynamics/1("sp_f ") -> Sum1/1
  Sum4/1 -> Scope2/1, Dynamics/1(sp_f)
  Sum1/1 -> Saturation/1
  w x (w x d)/1(w x ( w x d)) -> Sum/3
  Ab/1 -> Scope/1, Zero-Order Hold1/1
  Reshape1/1 -> Sum4/1
  Measurement bias/1 -> Sum4/2
  Product/1 -> Reshape1/1
  CG/1 -> Zero-Order Hold4/1
  pdot qdot rdot/1 -> Zero-Order Hold3/1
  p q r/1 -> Zero-Order Hold/1
  wdot x d/1 -> Sum/4
  Scale factors & Cross-coupling errors/1 -> Product/1
  Random bias/1 -> Sum1/2
  Saturation/1 -> Ameas/1
  Sum/1 -> Scope3/1, Product/2

== system Two_Attitude_Estimation_ekf/Sensors and preprocessing/IMU+altitude/Acc + Gyro/Three-axis Gyroscope ==
  p q r : Inport  Unit=rad/s  PortDimensions=3
  G's : Inport  Port=2  Unit=gn  PortDimensions=3
  Disallow CGS : UnitConfiguration  UnitSystemsStr=English,SI,SI (extended)  AllowAllUnitSystems=off
  Dynamics : Subsystem
  Measurement bias : Constant  Value=g_bias
  Product : Product  Multiplication=Matrix(*)  SaturateOnIntegerOverflow=on  OutDataTypeStr=Inherit: Same as first input
  Product1 : Product  SaturateOnIntegerOverflow=on  OutDataTypeStr=Inherit: Same as first input
  Random bias : aerolibcommonsys/Tunable White Noise  pwr=g_pow  Ts=g_Ts  seed=g_seeds
      settings: SourceProductBaseCode=AE
  Saturation : Saturate  UpperLimit=g_sath  LowerLimit=g_satl
  "Scale factors & Cross-coupling errors " : Constant  Value=g_sf_cc
  Sum1 : Sum  Inputs=|++  SaturateOnIntegerOverflow=on
  Sum4 : Sum  Inputs=+++  SaturateOnIntegerOverflow=on
  Zero-Order Hold : ZeroOrderHold  SampleTime=g_Ts
  Zero-Order Hold1 : ZeroOrderHold  SampleTime=g_Ts
  g-sensitive bias : Constant  Value=g_sen
  (p q r)_meas : Outport  Unit=rad/s  PortDimensions=3  VectorParamsAs1DForOutWhenUnconnected=off
  wires:
  Zero-Order Hold1/1 -> Product1/1
  Zero-Order Hold/1 -> Product/2
  Product1/1 -> Sum4/3
  Dynamics/1("p q r ") -> Sum1/1
  G's/1 -> Zero-Order Hold1/1
  Sum1/1 -> Saturation/1
  g-sensitive bias/1 -> Product1/2
  p q r/1 -> Zero-Order Hold/1
  Saturation/1 -> (p q r)_meas/1
  Random bias/1 -> Sum1/2
  "Scale factors & Cross-coupling errors "/1 -> Product/1
  Sum4/1 -> Dynamics/1(p q r)
  Product/1 -> Sum4/1
  Measurement bias/1 -> Sum4/2

== system Two_Attitude_Estimation_ekf/Control allocation and motor control/Ideal Actuators with allocation/Perfect actuators/Motor Control/w_MUX ==
  W_CMD : Inport
  W : Inport  Port=2
  Demux1 : Demux
  Demux2 : Demux
  Mux{,1..3} (4 alike) : Mux  Inputs=2
  w1 : Outport  VectorParamsAs1DForOutWhenUnconnected=off
  w2 : Outport  Port=2  VectorParamsAs1DForOutWhenUnconnected=off
  w3 : Outport  Port=3  VectorParamsAs1DForOutWhenUnconnected=off
  w4 : Outport  Port=4  VectorParamsAs1DForOutWhenUnconnected=off
  wires:
  W_CMD/1 -> Demux2/1
  W/1 -> Demux1/1
  Mux/1 -> w1/1
  Mux1/1 -> w2/1
  Mux3/1 -> w4/1
  Mux2/1 -> w3/1
  Demux2/1 -> Mux/1
  Demux2/2 -> Mux1/1
  Demux2/3 -> Mux2/1
  Demux2/4 -> Mux3/1
  Demux1/1 -> Mux/2
  Demux1/2 -> Mux1/2
  Demux1/3 -> Mux2/2
  Demux1/4 -> Mux3/2

== system Two_Attitude_Estimation_ekf/Sensors and preprocessing/IMU+altitude/Acc + Gyro/Three-axis Accelerometer/Dynamics ==
  sp_f : Inport
  Constant : Constant  Value=dtype_a
  No Dynamics : Subsystem
  Second-order Dynamics : aerolibnavsys/Transfer Fcn (D)  wn=w_a  zn=z_a  ts=a_Ts
      settings: SourceProductBaseCode=AE
  Switch : Switch  Threshold=0.5
  "sp_f " : Outport  VectorParamsAs1DForOutWhenUnconnected=off
  wires:
  Constant/1 -> Switch/2
  Switch/1 -> "sp_f "/1
  Second-order Dynamics/1 -> Switch/1
  No Dynamics/1(Out1) -> Switch/3
  sp_f/1 -> Second-order Dynamics/1, No Dynamics/1(In1)

== system Two_Attitude_Estimation_ekf/Sensors and preprocessing/IMU+altitude/Acc + Gyro/Three-axis Accelerometer/w x (w x d) ==
  "p q r " : Inport
  distance : Inport  Port=2
  w x (w x d) : sharedutil/3x3 Cross Product  aMode=aMode
      settings: SourceProductBaseCode=AE,PW,DR,MT,UV,VE
  w x d : sharedutil/3x3 Cross Product  aMode=aMode
      settings: SourceProductBaseCode=AE,PW,DR,MT,UV,VE
  w x ( w x d) : Outport  VectorParamsAs1DForOutWhenUnconnected=off
  wires:
  "p q r "/1 -> w x (w x d)/1, w x d/1
  w x d/1 -> w x (w x d)/2
  distance/1 -> w x d/2
  w x (w x d)/1 -> w x ( w x d)/1

== system Two_Attitude_Estimation_ekf/Sensors and preprocessing/IMU+altitude/Acc + Gyro/Three-axis Gyroscope/Dynamics ==
  p q r : Inport
  Constant : Constant  Value=dtype_g
  No Dynamics : Subsystem
  Second-order Dynamics : aerolibnavsys/Transfer Fcn (D)  wn=w_g  zn=z_g  ts=g_Ts
      settings: SourceProductBaseCode=AE
  Switch : Switch  Threshold=0.5
  "p q r " : Outport  VectorParamsAs1DForOutWhenUnconnected=off
  wires:
  p q r/1 -> Second-order Dynamics/1, No Dynamics/1(In1)
  No Dynamics/1(Out1) -> Switch/3
  Second-order Dynamics/1 -> Switch/1
  Switch/1 -> "p q r "/1
  Constant/1 -> Switch/2

== system Two_Attitude_Estimation_ekf/Sensors and preprocessing/IMU+altitude/Acc + Gyro/Three-axis Accelerometer/Dynamics/No Dynamics ==
  In1 : Inport
  Out1 : Outport  VectorParamsAs1DForOutWhenUnconnected=off
  wires:
  In1/1 -> Out1/1

== system Two_Attitude_Estimation_ekf/Sensors and preprocessing/IMU+altitude/Acc + Gyro/Three-axis Gyroscope/Dynamics/No Dynamics ==
  In1 : Inport
  Out1 : Outport  VectorParamsAs1DForOutWhenUnconnected=off
  wires:
  In1/1 -> Out1/1

== matlab function Two_Attitude_Estimation_ekf/State estimation/Measurement Jacobian ==
  data: x input; u input; H output
function H = calc_H(x,u)
% Jacobian of measurement model 
% Inputs:
%    xk - States x[k]
%    u - reference acc and mag vectors
ref_acc = u(1:3);
ref_mag = u(4:6);

% get current attitude quaternion
q0    = x(1);
q1    = x(2);
q2    = x(3);
q3    = x(4);

g = ref_acc(3);
M = ref_mag(1);

h_acc = 2*g*[
                -q2  q3 -q0 q1;
                 q1 q0   q3 q2;
                 q0 -q1 -q2 q3;
             ];
h_mag = 2*M*[
                 q0  q1 -q2 -q3;
                -q3  q2  q1 -q0;
                 q2  q3  q0  q1;
             ];         


H = [
    h_acc zeros(3);
    h_mag zeros(3);
    ];

== matlab function Two_Attitude_Estimation_ekf/Quad_EOM/Integrate_quaternion/MATLAB Function2 ==
  data: R input; phi output; theta output; psi output
function [phi,theta,psi] = euler_from_rot(R)
% Get Euler angles from rotation matrix (wolrd to body rotation matrix)
%NOTE:  this is bRg ... and NOT gRb

phi   = atan2(R(2,3),R(3,3));
theta = -asin(R(1,3));
psi   = atan2(R(1,2), R(1,1));
end

== matlab function Two_Attitude_Estimation_ekf/Control allocation and motor control/Ideal Actuators with allocation/Perfect actuators/Allocation matrix (motor speed to twist) ==
  data: L input; Thrust output; kt input; km input; w2_col input; M_x output; M_y output; M_z output
function [Thrust, M_x, M_y, M_z] = mixer(L, kt, km, w2_col)
%#codegen



    % construct the co-efficient matrix:
    %  T = C * w^2
    
%     C = [
%         kt  ,   kt   ,   kt  ,   kt  ;
%         0   , -L*kt  ,   0   , L*kt  ;
%        L*kt ,   0    , -L*kt ,   0   ;
%         km ,   -km   ,  km  ,   -km  ;
%     ];

    C = [
        -kt  ,   -kt  ,   -kt ,   -kt  ;
        0    , -L*kt   ,   0   , L*kt  ;
       L*kt ,   0    , -L*kt  ,   0   ;
        -km  ,   km   ,  -km  ,   km  ;
    ];

    % solve for the FM_col
    %   FM_col = [Thrust, M_x, M_y, M_z].' ;
    
    FM_col  =  C * w2_col;
    
    Thrust  =  FM_col(1);
    M_x     =  FM_col(2);
    M_y     =  FM_col(3);
    M_z     =  FM_col(4);
    
end

== matlab function Two_Attitude_Estimation_ekf/Quad_EOM/Integrate_quaternion/calc_bRg ==
  data: q input double size=[4, 1]; bRg output double size=[3 3]
function bRg = quat2dcm(q)
% convert quaternion to DCM
% the DCM represent coordinate transformation of a vector in inertial axes
% into body axes (bRg)

% VERY SLOW in SIMULINK

    q0    = q(1);
    qx    = q(2);
    qy    = q(3);
    qz    = q(4);
    
    C_11  = qx^2 + q0^2 - qy^2 - qz^2;
    C_12  = 2*(qx*qy + qz*q0);
    C_13  = 2*(qx*qz - qy*q0);
       
    C_21  = 2*(qx*qy - qz*q0);
    C_22  = qy^2 + q0^2 - qx^2 - qz^2;
    C_23  = 2*(qy*qz + qx*q0);
    
    C_31  = 2*(qx*qz + qy*q0);
    C_32  = 2*(qy*qz - qx*q0);
    C_33  = qz^2 + q0^2 - qx^2 - qy^2;
    
    
    bRg = [ C_11, C_12, C_13;
            C_21, C_22, C_23;
            C_31, C_32, C_33; ];   


end

== matlab function Two_Attitude_Estimation_ekf/Quad_EOM/Integrate_quaternion/calc_q_DOT ==
  data: q input double size=[4, 1]; q_dot output double size=[4 1]; wb input double size=[3, 1]
function q_dot = q_dot_from_rates(q, wb)
% angular rates are related to quaternion derivative by:
% note: this transformation is in body-fixed frame (body rates and
% quaternion in body-fixed frame)
% q_dot  = 0.5 * W^T * wb;
% 
% W = 
%    [-q1,  q0,  q3, -q2]
%    [-q2, -q3,  q0,  q1]
%    [-q3,  q2, -q1,  q0]
% W_transpose = 
%             [-q1, -q2, -q3]
%             [ q0, -q3,  q2]
%             [ q3,  q0, -q1]
%             [-q2,  q1,  q0]

q0     = q(1);
q1     = q(2);
q2     = q(3);
q3     = q(4);

W_transpose =  [
                 -q1, -q2, -q3;
                  q0, -q3,  q2;
                  q3,  q0, -q1;
                 -q2,  q1,  q0;
                 ];

wb = wb(:);

q_dot  = 0.5 * W_transpose * wb;

end

== matlab function Two_Attitude_Estimation_ekf/State estimation/Extended Kalman Filter With Analytical Jacobian/Output/MATLAB Function ==
  data: S input; P output
function P = fcn(S)
    
    % Get back Covariance from Square-root Covariance
    P = S*S';
    
end

== matlab function Two_Attitude_Estimation_ekf/State estimation/Extended Kalman Filter With Analytical Jacobian/Predict/Predict ==
  settings: updateMethod=DISCRETE  sampleTime=SampleTime
  data: x input; xNew output; P input; Q input; uState input; unused input; P output; pS parameter
function [xNew,P] = fcn(x,P,Q,uState,~,pS)
% ekfCorrect Prediction step for EKF
%
%   Copyright 2016-2017 The MathWorks, Inc.

%#codegen

% If process noise is time-varying then compute square-root
% factorization.
if pS.HasTimeVaryingQ
   Q = matlabshared.tracking.internal.svdPSD(Q);
end

% Construct fcn handles
if pS.IsSimulinkFcn
    StateTransitionJacobianFcnH_SL = str2func(pS.FcnName);
    if pS.HasAdditiveNoise
        StateTransitionFcnH = @(fState)StateTransitionJacobianFcnH_SL(fState);
    else
        StateTransitionFcnH = @(fState,fProcNoise)StateTransitionJacobianFcnH_SL(fState,fProcNoise);
    end
else
    StateTransitionFcnH = str2func(pS.FcnName);
end
if pS.HasJacobian
    if pS.IsSimulinkFcn
        StateTransitionJacobianFcnH_SL = str2func(pS.JacobianFcnName);
        if pS.HasAdditiveNoise
            StateTransitionJacobianFcnH = @(fState)StateTransitionJacobianFcnH_SL(fState);
        else
            StateTransitionJacobianFcnH = @(fState,fProcNoise)StateTransitionJacobianFcnH_SL(fState,fProcNoise);
        end
    else
        StateTransitionJacobianFcnH = str2func(pS.JacobianFcnName);
    end
else
    StateTransitionJacobianFcnH = [];
end

switch pS.NumberOfExtraArgumentInports
    case 0
        extraArgs = {};
    case 1
        extraArgs = {uState};
    otherwise
        assert(false);
end

% Check if dimensions and type of State and Jacobian are correct
if pS.HasAdditiveNoise
   % Additive noise
   
   % StateTransitionFcn
   xTry = StateTransitionFcnH(x, extraArgs{:});
   
   if pS.IsSimulinkFcn
      hasError = any(size(x) ~= size(xTry));
   else
      hasError = any(size(x) ~= size(xTry)) || ~isa(xTry, class(x));
   end
   
   coder.internal.errorIf(...
      hasError,...
      'shared_tracking:ExtendedKalmanFilter:StateNonMatchingSizeOrClass',...
      'StateTransitionFcn', 'State', numel(x));
   
   if pS.HasJacobian
      % Jacobian
      F = StateTransitionJacobianFcnH(x, extraArgs{:});
      % F needs to be square
      isSizeNotCorrect = ~all(size(F) == numel(x));
      
      if pS.IsSimulinkFcn
         hasError = isSizeNotCorrect;
      else
         hasError = isSizeNotCorrect || ~isa(F, class(x));
      end
      
      coder.internal.errorIf(...
         hasError,...
         'shared_tracking:ExtendedKalmanFilter:StateTransitionJacobianNonMatchingSizeOrClass',...
         'StateTransitionJacobianFcn', numel(x));
   end
else
   % Non-additive noise
   
   % StateTransitionFcn
   xTry = StateTransitionFcnH(x, zeros(size(Q,1),1,'like',x),extraArgs{:});
   
   if pS.IsSimulinkFcn
      hasError = any(size(x) ~= size(xTry));
   else
      hasError = any(size(x) ~= size(xTry)) || ~isa(xTry, class(x));
   end
   
   coder.internal.errorIf(...
      hasError,...
      'shared_tracking:ExtendedKalmanFilter:StateNonMatchingSizeOrClass',...
      'StateTransitionFcn', 'State', numel(x))
   
   if pS.HasJacobian
      % Jacobian
      F = StateTransitionJacobianFcnH(x, zeros(size(Q,1),1,'like',x),extraArgs{:});
      % F needs to be square
      isSizeNotCorrect = ~all(size(F) == numel(x));
      
      if pS.IsSimulinkFcn
         hasError = isSizeNotCorrect;
      else
         hasError = isSizeNotCorrect || ~isa(F, class(x));
      end
       
      coder.internal.errorIf(...
         hasError,...
         'shared_tracking:ExtendedKalmanFilter:StateTransitionJacobianNonMatchingSizeOrClass',...
         'StateTransitionJacobianFcn', numel(x));
   end
end

xNew = zeros(size(x),'like',x); %#ok<PREALL>

if pS.HasAdditiveNoise
    [xNew,P] = matlabshared.tracking.internal.EKFPredictorAdditive.predict(...
        Q,x,P,StateTransitionFcnH,StateTransitionJacobianFcnH,extraArgs{:});
else    
    [xNew,P] = matlabshared.tracking.internal.EKFPredictorNonAdditive.predict(...
        Q,x,P,StateTransitionFcnH,StateTransitionJacobianFcnH,extraArgs{:});
end
end

== matlab function Two_Attitude_Estimation_ekf/State estimation/Extended Kalman Filter With Analytical Jacobian/Correct1/Correct ==
  settings: updateMethod=DISCRETE  sampleTime=SampleTime
  data: x input; xNew output; P input; P output; yMeas input; R input; uMeas input; blockOrdering input; pM parameter; blockOrdering output
function [xNew,P,blockOrdering] = fcn(x,P,yMeas,R,uMeas,blockOrdering,pM)
% ekfCorrect Correction step for EKF
%
%   Copyright 2016-2018 The MathWorks, Inc.

%#codegen

% If measurement noise is time-varying then compute square-root
% factorization.
if pM.HasTimeVaryingR
   R = matlabshared.tracking.internal.svdPSD(R);
end

% Construct the function handle for measurement fcn
if pM.IsSimulinkFcn
    MeasurementFcnH_SL = str2func(pM.FcnName);
    if pM.HasAdditiveNoise
        MeasurementFcnH = @(fState)MeasurementFcnH_SL(fState);
    else
        MeasurementFcnH = @(fState,fMeasNoise)MeasurementFcnH_SL(fState,fMeasNoise);
    end
else
    MeasurementFcnH = str2func(pM.FcnName);
end

% Construct the function handle for measurement Jacobian fcn
if pM.HasJacobian
    if pM.IsSimulinkFcn
        MeasurementJacobianFcnH_SL = str2func(pM.JacobianFcnName);
        if pM.HasAdditiveNoise
            MeasurementJacobianFcnH = @(fState)MeasurementJacobianFcnH_SL(fState);
        else
            MeasurementJacobianFcnH = @(fState,fMeasNoise)MeasurementJacobianFcnH_SL(fState,fMeasNoise);
        end
    else
        MeasurementJacobianFcnH = str2func(pM.JacobianFcnName);
    end
else
    MeasurementJacobianFcnH = [];
end

% Handle (optional) extra input arguments of the measurement & jacobian fcns
switch pM.NumberOfExtraArgumentInports
    case 0
        extraArgs = {};
    case 1
        extraArgs = {uMeas};
    otherwise
        assert(false);
end

% Construct the corrector, perform the update
if pM.HasAdditiveNoise
    ekfCorrector = matlabshared.tracking.internal.EKFCorrectorAdditive();
else
    ekfCorrector = matlabshared.tracking.internal.EKFCorrectorNonAdditive();
end

% Check if dimensions and type of Measurement and Jacobian are correct
if pM.HasAdditiveNoise
   % Additive noise
   
   % MeasurementFcn
   ztry = MeasurementFcnH(x, extraArgs{:});
   
   if pM.IsSimulinkFcn
      hasError = (numel(ztry) ~= numel(yMeas));
   else
      hasError = (numel(ztry) ~= numel(yMeas)) || ~isa(ztry, class(x));
   end
   
   coder.internal.errorIf(...
      hasError,...
      'shared_tracking:ExtendedKalmanFilter:MeasurementNonMatchingSizeOrClass',...
      'MeasurementFcn');
   
   if pM.HasJacobian
      % MeasurementJacobianFcn
      Htry = MeasurementJacobianFcnH(x, extraArgs{:});
      isSizeNotCorrect = numel(yMeas) ~= size(Htry,1) || numel(x) ~= size(Htry,2);
      
      if pM.IsSimulinkFcn
         hasError = isSizeNotCorrect;
      else
         hasError = isSizeNotCorrect || ~isa(Htry, class(x));
      end
      
      coder.internal.errorIf(...
         hasError,...
         'shared_tracking:ExtendedKalmanFilter:MeasurementJacobianNonMatchingSizeOrClass',...
         'MeasurementJacobianFcn',numel(yMeas),numel(x));
   end   
else
   % Non-additive noise
   
   % MeasurementFcn
   ztry = MeasurementFcnH(...
      x, zeros(size(R,1),1,'like',x), ...
      extraArgs{:});   

   if pM.IsSimulinkFcn
      hasError = (numel(ztry) ~= numel(yMeas));
   else
      hasError = (numel(ztry) ~= numel(yMeas)) || ~isa(ztry, class(x));
   end
   
   coder.internal.errorIf(...
      hasError,...
      'shared_tracking:ExtendedKalmanFilter:MeasurementNonMatchingSizeOrClass',...
      'MeasurementFcn');
   
   if pM.HasJacobian
      % MeasurementJacobianFcn
      Htry = MeasurementJacobianFcnH(...
         x, zeros(size(R,1),1,'like',x), ...
         extraArgs{:});
      
      isSizeNotCorrect = numel(yMeas) ~= size(Htry,1) || numel(x) ~= size(Htry,2);     
      
      if pM.IsSimulinkFcn
         hasError = isSizeNotCorrect;
      else
         hasError = isSizeNotCorrect || ~isa(Htry, class(x));
      end
      
      coder.internal.errorIf(...
         hasError,...
         'shared_tracking:ExtendedKalmanFilter:MeasurementJacobianNonMatchingSizeOrClass',...
         'MeasurementJacobianFcn',numel(yMeas),numel(x));
   end
end

xNew = zeros(size(x),'like',x); %#ok<PREALL>

[xNew,P] = ekfCorrector.correct(...
        yMeas,R,x,P,MeasurementFcnH,MeasurementJacobianFcnH,extraArgs{:});
end

== matlab function Two_Attitude_Estimation_ekf/Quad with sensors+estimator/Attitude representation/Calc Euler_rates/euler_rates ==
  data: phi_t input; euler_rates output; theta_t input; p input; q input; r input
function euler_rates = euler_rates(phi_t,theta_t,p,q,r)
%#codegen

%    This function was generated by the Symbolic Math Toolbox version 8.7.
%    04-Nov-2022 08:55:55

euler_rates = [(p.*cos(theta_t)+r.*cos(phi_t).*sin(theta_t)+q.*sin(phi_t).*sin(theta_t))./cos(theta_t);q.*cos(phi_t)-r.*sin(phi_t);(r.*cos(phi_t)+q.*sin(phi_t))./cos(theta_t)];

== matlab function Two_Attitude_Estimation_ekf/Quad with sensors+estimator/Attitude representation/MATLAB Function2 ==
  data: R input; phi output; theta output; psi output
function [phi,theta,psi] = euler_from_rot(R)
% Get Euler angles from rotation matrix (wolrd to body rotation matrix)
%NOTE:  this is bRg ... and NOT gRb

phi   = atan2(R(2,3),R(3,3));
theta = -asin(R(1,3));
psi   = atan2(R(1,2), R(1,1));
end

== matlab function Two_Attitude_Estimation_ekf/Quad with sensors+estimator/Attitude representation/calc_bRg ==
  data: q input double size=[4, 1]; bRg output double size=[3 3]
function bRg = quat2dcm(q)
% convert quaternion to DCM
% the DCM represent coordinate transformation of a vector in inertial axes
% into body axes (bRg)

% VERY SLOW in SIMULINK

    q0    = q(1);
    qx    = q(2);
    qy    = q(3);
    qz    = q(4);
    
    C_11  = qx^2 + q0^2 - qy^2 - qz^2;
    C_12  = 2*(qx*qy + qz*q0);
    C_13  = 2*(qx*qz - qy*q0);
       
    C_21  = 2*(qx*qy - qz*q0);
    C_22  = qy^2 + q0^2 - qx^2 - qz^2;
    C_23  = 2*(qy*qz + qx*q0);
    
    C_31  = 2*(qx*qz + qy*q0);
    C_32  = 2*(qy*qz - qx*q0);
    C_33  = qz^2 + q0^2 - qx^2 - qy^2;
    
    
    bRg = [ C_11, C_12, C_13;
            C_21, C_22, C_23;
            C_31, C_32, C_33;   ];   


end

== matlab function Two_Attitude_Estimation_ekf/State estimation/MATLAB Function ==
  data: u input; y output; v input
function y = orientationError(u,v)
%ORIENTATIONERROR Compute the quaternion distance in degrees

%   Copyright 2019 The MathWorks, Inc.   

y = rad2deg(dist(quaternion(u'), quaternion(v')));

== matlab function Two_Attitude_Estimation_ekf/Quad with sensors/Integrate_quaternion/Calc Euler_rates/euler_rates ==
  data: phi_t input; euler_rates output; theta_t input; p input; q input; r input
function euler_rates = euler_rates(phi_t,theta_t,p,q,r)
%#codegen

%    This function was generated by the Symbolic Math Toolbox version 8.7.
%    04-Nov-2022 08:55:55

euler_rates = [(p.*cos(theta_t)+r.*cos(phi_t).*sin(theta_t)+q.*sin(phi_t).*sin(theta_t))./cos(theta_t);q.*cos(phi_t)-r.*sin(phi_t);(r.*cos(phi_t)+q.*sin(phi_t))./cos(theta_t)];

== matlab function Two_Attitude_Estimation_ekf/Quad with sensors/Integrate_quaternion/MATLAB Function2 ==
  data: R input; phi output; theta output; psi output
function [phi,theta,psi] = euler_from_rot(R)
% Get Euler angles from rotation matrix (wolrd to body rotation matrix)
%NOTE:  this is bRg ... and NOT gRb

phi   = atan2(R(2,3),R(3,3));
theta = -asin(R(1,3));
psi   = atan2(R(1,2), R(1,1));
end

== matlab function Two_Attitude_Estimation_ekf/Quad with sensors/Integrate_quaternion/NORMLIZE_occasionally/Adjust_to_UNITY/MATLAB Function ==
  data: change_signal input double size=1; q output; q_in input double size=[4 1]; mag_of_q output
function [q, mag_of_q] = fcn(change_signal, q_in)

if(change_signal > 0.5)
    q = q_in / norm(q_in);
else
    q = q_in;
end

mag_of_q = norm(q);

end

== matlab function Two_Attitude_Estimation_ekf/Quad_EOM/Integrate_quaternion/NORMLIZE_occasionally/Adjust_to_UNITY/MATLAB Function ==
  data: change_signal input double size=1; q output; q_in input double size=[4 1]; mag_of_q output
function [q, mag_of_q] = fcn(change_signal, q_in)

if(change_signal > 0.5)
    q = q_in / norm(q_in);
else
    q = q_in;
end

mag_of_q = norm(q);

end

== matlab function Two_Attitude_Estimation_ekf/Quad with sensors/Integrate_quaternion/calc_bRg ==
  data: q input double size=[4, 1]; bRg output double size=[3 3]
function bRg = quat2dcm(q)
% convert quaternion to DCM
% the DCM represent coordinate transformation of a vector in inertial axes
% into body axes (bRg)

% VERY SLOW in SIMULINK

    q0    = q(1);
    qx    = q(2);
    qy    = q(3);
    qz    = q(4);
    
    C_11  = qx^2 + q0^2 - qy^2 - qz^2;
    C_12  = 2*(qx*qy + qz*q0);
    C_13  = 2*(qx*qz - qy*q0);
       
    C_21  = 2*(qx*qy - qz*q0);
    C_22  = qy^2 + q0^2 - qx^2 - qz^2;
    C_23  = 2*(qy*qz + qx*q0);
    
    C_31  = 2*(qx*qz + qy*q0);
    C_32  = 2*(qy*qz - qx*q0);
    C_33  = qz^2 + q0^2 - qx^2 - qy^2;
    
    
    bRg = [ C_11, C_12, C_13;
            C_21, C_22, C_23;
            C_31, C_32, C_33;   ];   


end

== matlab function Two_Attitude_Estimation_ekf/Quad with sensors/Integrate_quaternion/calc_q_DOT ==
  data: q input double size=[4, 1]; q_dot output double size=[4 1]; wb input double size=[3, 1]
function q_dot = q_dot_from_rates(q, wb)
% angular rates are related to quaternion derivative by:
% note: this transformation is in body-fixed frame (body rates and
% quaternion in body-fixed frame)
% q_dot  = 0.5 * W^T * wb;
% 
% W = 
%    [-q1,  q0,  q3, -q2]
%    [-q2, -q3,  q0,  q1]
%    [-q3,  q2, -q1,  q0]
% W_transpose = 
%             [-q1, -q2, -q3]
%             [ q0, -q3,  q2]
%             [ q3,  q0, -q1]
%             [-q2,  q1,  q0]

q0     = q(1);
q1     = q(2);
q2     = q(3);
q3     = q(4);

W_transpose =  [
                 -q1, -q2, -q3;
                  q0, -q3,  q2;
                  q3,  q0, -q1;
                 -q2,  q1,  q0;
                 ];

wb = wb(:);

q_dot  = 0.5 * W_transpose * wb;

end

== matlab function Two_Attitude_Estimation_ekf/Sensors and preprocessing/IMU+altitude/Compare yaw from mag and actual one ==
  data: acc_vec input; yaw output; mag_vec input
function yaw = accMag2yaw(acc_vec,mag_vec)
% Estimate yaw from accelerometer and magnetometer
% acc will estimate roll and pitch
% mag+roll+pitch will estimate yaw
% Note: this assumes no movement and acceleration is only due to gravity
% note: this doesn't work when roll is pi/2 (singular)
ax = acc_vec(1);
ay = acc_vec(2);
az = acc_vec(3);
mx = mag_vec(1);
my = mag_vec(2);
mz = mag_vec(3);


g = 9.8100;
roll = asin(-ax/g);
pitch = atan2(az ,ay);
yaw = atan2(mx,cos(pitch)*(mz*sin(roll)-my*cos(roll)))-pi/2;


%% another approach
% roll = atan2 (az ,ay);
% az2 = ay * sin ( roll ) + az * cos ( roll );
% pitch = atan2 ( az2, - ax );
% my2 = mz * sin ( roll ) - my * cos ( roll );
% mz2 = my * sin ( roll ) + mz * cos ( roll );
% mx3 = mx * cos ( pitch )+ mz2 * sin ( pitch );
% yaw = atan2 ( mx3,my2 )-pi/2;

== matlab function Two_Attitude_Estimation_ekf/Quad with sensors/Process model testing/MATLAB Function ==
  data: u input; y output; v input
function y = orientationError(u,v)
%ORIENTATIONERROR Compute the quaternion distance in degrees

%   Copyright 2019 The MathWorks, Inc.   

y = rad2deg(dist(quaternion(u'), quaternion(v')));

== matlab function Two_Attitude_Estimation_ekf/Quad with sensors/Process model testing/Predict xk+1 ==
  data: x input; xk output; w input
function xk = process_model(x,w)
% process model of quaternion attitude as per quaternion integration
% w is the body angular rates measurement from gyro 

% q_dot=0.5*S(w)*q=0.5*S(q)*w
% the gyro bias is added resulting in 
% q_dot=0.5*S(w-b)*q=0.5*S(q)*(w-b)
% Converting to matrix form and using first order integration
% x(k+1) = F*x(k)+B*w
% where w is coming from gyro measurements
% note that this is a linear model


% q_dot  = 0.5 * S(w-b) * q;

Ts = 0.001; % update interval
q0     = x(1);
q1     = x(2);
q2     = x(3);
q3     = x(4);

Sq =  [
                -q1, -q2, -q3;
                 q0, -q3,  q2;
                 q3,  q0, -q1;
                -q2,  q1,  q0;
       ];



A = [
        eye(4)       -(Ts/2)*Sq;
        zeros(3,4)   eye(3);
    ];

B = [
        (Ts/2)*Sq;
        zeros(3);
    ];

w = w(:);
xk  = A*x+B*w;

% normalize quaternion
%xk(1:4) =  quaternion(xk(1:4)').normalize().compact;
xk(1:4) = xk(1:4)/norm(xk(1:4));


%%  ignoring bias
% xk = zeros(7,1);
% q_dot  = 0.5 * Sq * w;
% xk(1:4) = [q0;q1;q2;q3]+q_dot*Ts; % integrate
% xk(1:4) = xk(1:4)/norm(xk(1:4));
end

== matlab function Two_Attitude_Estimation_ekf/Attitude control/MATLAB Function1 ==
  data: q0 input; y output
function y = sign(q0)
if q0>=0
    y = 1;
else
    y = -1;
end

== matlab function Two_Attitude_Estimation_ekf/Control allocation and motor control/Ideal Actuators with allocation/Control allocation/FM_to_w2 ==
  data: L input; w2_cmd output; kt input; km input; Thrust input; M_x input; M_y input; M_z input
function w2_cmd = control_allocation(L, kt, km, Thrust, M_x, M_y, M_z)
%#codegen

    % construct the co-efficient matrix:
    %  F_and_M = C * w^2
    %
    % C = [
    %     kt  ,   kt   ,   kt  ,   kt  ;
    %     0   , -L*kt  ,   0   , L*kt  ;
    %    L*kt ,   0    , -L*kt ,   0   ;
    %     km ,   -km   ,  km  ,   -km  ;
    % ];

    % used Symbolic toolbox to compute inv(C)
%     C_inv = [
%                 1/(4*kt),          0 ,  1/(2*L*kt),  1/(4*km);
%                 1/(4*kt), -1/(2*L*kt),           0,  -1/(4*km); 
%                 1/(4*kt),          0 , -1/(2*L*kt),  1/(4*km);
%                 1/(4*kt), 1/(2*L*kt) ,          0 ,  -1/(4*km);
%              ];
         
    C_inv = [
             -1/(4*kt),            0,   1/(2*L*kt), -1/(4*km);
             -1/(4*kt),  -1/(2*L*kt),            0,  1/(4*km);
             -1/(4*kt),            0,  -1/(2*L*kt), -1/(4*km);
             -1/(4*kt),   1/(2*L*kt),            0,  1/(4*km);
            ];        
    % solve for the w^2 vec
    F_and_M_col = [Thrust, M_x, M_y, M_z].' ;

    w2_cmd = C_inv * F_and_M_col;
   
end

== matlab function Two_Attitude_Estimation_ekf/Position+Velocity Control/Velocity PID Controller/MATLAB Function ==
  data: Tmax input; tilt_max input; Tx input; Tx output; Ty input; Tz input; Ty output
function [Tx, Ty] = limit_tilt( Tmax, tilt_max, Tx, Ty, Tz)
% horizontal thrust magnituide at max tilt angle
T_hor = abs(Tz)*tan(tilt_max);
% maximum availble horizontal thrust magnituide 
T_hor_max = sqrt(abs(Tmax^2-Tz^2));
% limit horizontal thrust magnituide to max available
T_hor = min(T_hor,T_hor_max);

% saturate horizonal thrust components Tx,Ty if exceed T_hor
if Tx^2+Ty^2 > T_hor
   T_xy = norm([Tx,Ty]);
   Tx = (Tx/T_xy)*T_hor;
   Ty = (Ty/T_xy)*T_hor;

else
   Tx = Tx;
   Ty = Ty;

end

== matlab function Two_Attitude_Estimation_ekf/Thrust to attitude/MATLAB Function4 ==
  data: thrust_sp input; R_sp output; yaw_sp input; thrust_mag output
function [R_sp,thrust_mag] = thurst2attitude(thrust_sp, yaw_sp)
% Create Full Desired Quaternion Based on Thrust Setpoint and Desired Yaw Angle
% from px4
    % Desired body_z axis direction
    body_z = -thrust_sp/norm(thrust_sp);

    % Vector of desired Yaw direction in XY plane, rotated by pi/2 (fake body_y axis)
    y_C = [-sin(yaw_sp), cos(yaw_sp), 0.0].';

    % Desired body_x axis direction
    body_x = cross(y_C, body_z);
    body_x = body_x/norm(body_x); % normalize

    % Desired body_y axis direction
    body_y = cross(body_z, body_x);

    % Desired rotation matrix
    R_sp = [body_x, body_y, body_z].';

    thrust_mag = -norm(thrust_sp);

== matlab function Two_Attitude_Estimation_ekf/State estimation/Z-H(x) innovation/MATLAB Function1 ==
  data: P input; S output; H input; R input
function S = innov_cov(P,H,R)
H_t = H';
S = H*P*H_t+R;

== matlab function Two_Attitude_Estimation_ekf/Quad_EOM/Integrate_quaternion/Calc Euler_rates/euler_rates ==
  data: phi_t input; euler_rates output; theta_t input; p input; q input; r input
function euler_rates = euler_rates(phi_t,theta_t,p,q,r)
%#codegen

%    This function was generated by the Symbolic Math Toolbox version 8.7.
%    04-Nov-2022 08:55:55

euler_rates = [(p.*cos(theta_t)+r.*cos(phi_t).*sin(theta_t)+q.*sin(phi_t).*sin(theta_t))./cos(theta_t);q.*cos(phi_t)-r.*sin(phi_t);(r.*cos(phi_t)+q.*sin(phi_t))./cos(theta_t)];

== matlab function Two_Attitude_Estimation_ekf/State estimation/measure xk+1 ==
  data: x input; y output; u input
function y = measurement_model(x,u)
% measurement model, assuming additive noise
% z[k] = h(x[k],u[k])
% sensors: magnetormeter and accelerometer
% u: references for mag (site-specific mag field from calibration) and acc (gravity vector)
ref_acc = u(1:3);
ref_mag = u(4:6);

% get current attitude quaternion
q0    = x(1);
qx    = x(2);
qy    = x(3);
qz    = x(4);

% convert quaternion to DCM (body to world)
C_11  = qx^2 + q0^2 - qy^2 - qz^2;
C_12  = 2*(qx*qy + qz*q0);
C_13  = 2*(qx*qz - qy*q0);

C_21  = 2*(qx*qy - qz*q0);
C_22  = qy^2 + q0^2 - qx^2 - qz^2;
C_23  = 2*(qy*qz + qx*q0);

C_31  = 2*(qx*qz + qy*q0);
C_32  = 2*(qy*qz - qx*q0);
C_33  = qz^2 + q0^2 - qx^2 - qy^2;
bRg = [ C_11, C_12, C_13;
        C_21, C_22, C_23;
        C_31, C_32, C_33; ];   

% acc measurement model
z_acc = bRg*ref_acc ;

% mag measurement model
z_mag = bRg*ref_mag;
y = [z_acc;z_mag];
